simulink model "robot_stand"  (R2014b)
settings: Solver=ode45  StartTime=0.0  StopTime=10  FixedStep=1e-4  RelTol=1e-3
values from neighbouring files (symbols this model uses):
  robot_floor_friction_coeff = 0.6    [robot_init.m]
  robot_floor_position_gain = -1e5    (= -100000)    [robot_init.m]
  robot_floor_speed_gain = -1e3    (= -1000)    [robot_init.m]
  robot_gravity = [0 0 -9.80665]    [robot_init.m]
undefined symbols (not defined in the file or in its folder): CM730_acc_center, CM730_acc_gain, CM730_default, CM730_gyro_center, CM730_gyro_gain, CM730_sample_time, FSR_max, FSR_no_load, FSR_sample_time, FSR_scale, MX28_default, MX28_inertia, MX28_Te, X, Y, Z
libraries: sm_lib x158, fl_lib x128, nesl_utility x77
(part 1 of 6)
settings Model: BufferReuse=off  Creator=florent  LastModifiedBy=florent
settings DataIOCC: LimitDataPoints=off  SaveOutput=off  SignalLogging=off  DSMLogging=off  SaveTime=off
settings OptimizationCC: OptimizeBlockIOStorage=off  BufferReuse=off  GlobalBufferReuse=off  ExpressionFolding=off  LocalBlockOutputs=off
settings DebuggingCC: StateNameClashWarn=warning
settings DiagnosticsConfigSet: SimMechanicsConflictingReferenceFrames=none

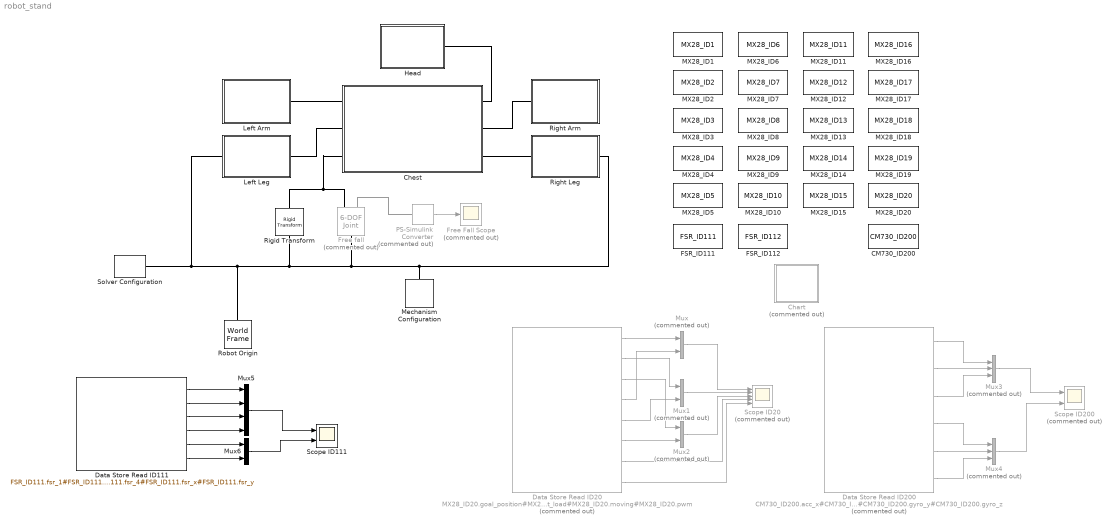
== system robot_stand ==
  CM730_ID200 : DataStoreMemory  DataStoreName=CM730_ID200  WriteAfterWriteMsg=error  InitialValue=CM730_default  VectorParams1D=off  OutDataTypeStr=Bus: CM730_bus
  Chart : Stateflow chart  Commented=on  TreatAsAtomicUnit=on
  Chest : Subsystem
      mask init:
      | [ModelDir,~,~] = fileparts(which(gcs));
      | 
      | Block = [gcb '/Solid'];
      | STLFileName = [ModelDir filesep 'STL' filesep 'Chest.STL'];
      | if ~strcmp(get_param(Block,'ExtGeomFileName'),STLFileName)
      |     set_param(Block,'ExtGeomFileName',STLFileName);
      | end
  Data Store Read ID111 : DataStoreRead  DataStoreName=FSR_ID111  SampleTime=MX28_Te  DataStoreElements=FSR_ID111.fsr_1#FSR_ID111.fsr_2#FSR_ID111.fsr_3#FSR_ID111.fsr_4#FSR_ID111.fsr_x#FSR_ID111.fsr_y
  Data Store Read ID20 : DataStoreRead  Commented=on  DataStoreName=MX28_ID20  SampleTime=MX28_Te  DataStoreElements=MX28_ID20.goal_position#MX28_ID20.moving_speed#MX28_ID20.torque_limit#MX28_ID20.present_position#MX28_ID20.present_speed#MX28_ID20.present_load#MX28_ID20.moving#MX28_ID20.pwm
  Data Store Read ID200 : DataStoreRead  Commented=on  DataStoreName=CM730_ID200  SampleTime=MX28_Te  DataStoreElements=CM730_ID200.acc_x#CM730_ID200.acc_y#CM730_ID200.acc_z#CM730_ID200.gyro_x#CM730_ID200.gyro_y#CM730_ID200.gyro_z
  FSR_ID111 : DataStoreMemory  DataStoreName=FSR_ID111  WriteAfterWriteMsg=error  InitialValue=FSR_default  VectorParams1D=off  OutDataTypeStr=Bus: FSR_bus
  FSR_ID112 : DataStoreMemory  DataStoreName=FSR_ID112  WriteAfterWriteMsg=error  InitialValue=FSR_default  VectorParams1D=off  OutDataTypeStr=Bus: FSR_bus
  Free Fall Scope : Scope  Commented=on
      settings: YMin=0.3418  YMax=0.34205  SaveName=ScopeData2
  Free fall : sm_lib/Joints/6-DOF Joint  Commented=on  SenseConstraintForce=off  SenseConstraintForceX=off  SenseConstraintForceY=off  SenseConstraintForceZ=off  SenseConstraintTorque=off  SenseConstraintTorqueX=off  SenseConstraintTorqueY=off  SenseConstraintTorqueZ=off  SenseTotalForce=off  SenseTotalForceX=off  SenseTotalForceY=off  SenseTotalForceZ=off  SenseTotalTorque=off  SenseTotalTorqueX=off  SenseTotalTorqueY=off  SenseTotalTorqueZ=off  CompositeWrenchDir=FollowerOnBase  CompositeWrenchFrame=BaseFrame  PxEquilibriumPosition=0  PxEquilibriumPositionUnits=m  PxSpringStiffness=0  PxSpringStiffnessUnits=N/m  PxDampingCoefficient=0  PxDampingCoefficientUnits=N/(m/s)  PxTorqueActuationMode=NoTorque  PxMotionActuationMode=ComputedMotion  PxSensePosition=off  PxSenseVelocity=off  PxSenseAcceleration=off  PxSenseTorqueForce=off  PxPositionTargetValue=0  PxPositionTargetValueUnits=m  PxPositionTargetSpecify=off  PxPositionTargetPriority=High  PxVelocityTargetValue=0  PxVelocityTargetValueUnits=m/s  PxVelocityTargetSpecify=off  PxVelocityTargetPriority=High  PyEquilibriumPosition=0  PyEquilibriumPositionUnits=m  PySpringStiffness=0  PySpringStiffnessUnits=N/m  PyDampingCoefficient=0  PyDampingCoefficientUnits=N/(m/s)  PyTorqueActuationMode=NoTorque  PyMotionActuationMode=ComputedMotion  PySensePosition=off  PySenseVelocity=off  PySenseAcceleration=off  PySenseTorqueForce=off  PyPositionTargetValue=0  PyPositionTargetValueUnits=m  PyPositionTargetSpecify=off  PyPositionTargetPriority=High  PyVelocityTargetValue=0  PyVelocityTargetValueUnits=m/s  PyVelocityTargetSpecify=off  PyVelocityTargetPriority=High  PzEquilibriumPosition=0  PzEquilibriumPositionUnits=m  PzSpringStiffness=0  PzSpringStiffnessUnits=N/m  PzDampingCoefficient=0  PzDampingCoefficientUnits=N/(m/s)  PzTorqueActuationMode=NoTorque  PzMotionActuationMode=ComputedMotion  PzSensePosition=on  PzSenseVelocity=off  PzSenseAcceleration=off  PzSenseTorqueForce=off  PzPositionTargetValue=342  PzPositionTargetValueUnits=mm  PzPositionTargetSpecify=on  PzPositionTargetPriority=High  PzVelocityTargetValue=0  PzVelocityTargetValueUnits=m/s  PzVelocityTargetSpecify=off  PzVelocityTargetPriority=High  SphDefPosRotationMethod=None  SphDefPosRotationAngleUnits=deg  SphDefPosRotationStandardAxis=+Z  SphDefPosRotationAngle=0.0  SphDefPosRotationArbitraryAxis=[0 0 1]  SphDefPosFollAlignAxisA=+X  SphDefPosBaseAlignAxisA=+Y  SphDefPosFollAlignAxisB=+Y  SphDefPosBaseAlignAxisB=+Z  SphDefPosRotationMatrix=[1 0 0; 0 1 0; 0 0 1]  SphEqPosRotationMethod=None  SphEqPosRotationAngleUnits=deg  SphEqPosRotationStandardAxis=+Z  SphEqPosRotationAngle=0.0  SphEqPosRotationArbitraryAxis=[0 0 1]  SphEqPosFollAlignAxisA=+X  SphEqPosBaseAlignAxisA=+Y  SphEqPosFollAlignAxisB=+Y  SphEqPosBaseAlignAxisB=+Z  SphEqPosRotationMatrix=[1 0 0; 0 1 0; 0 0 1]  SphSpringStiffness=0  SphSpringStiffnessUnits=N*m/deg  SphDampingCoefficient=0  SphDampingCoefficientUnits=N*m/(deg/s)  SphActuateTorqueX=off  SphActuateTorqueY=off  SphActuateTorqueZ=off  SphActuateTorque=off  SphTorqueActuationMode=NoTorque  SphMotionActuationMode=ComputedMotion  SphActuationFrame=BaseFrame  SphSensePosition=off  SphSenseVelocityX=off  SphSenseVelocityY=off  SphSenseVelocityZ=off  SphSenseVelocity=off  SphSenseAccelerationX=off  SphSenseAccelerationY=off  SphSenseAccelerationZ=off  SphSenseAcceleration=off  SphSenseTorqueX=off  SphSenseTorqueY=off  SphSenseTorqueZ=off  SphSenseTorqueForce=off  SphSensingFrame=BaseFrame  SphPositionTargetRotationMethod=None  SphPositionTargetRotationAngleUnits=deg  SphPositionTargetRotationStandardAxis=+Z  SphPositionTargetRotationAngle=0.0  SphPositionTargetRotationArbitraryAxis=[0 0 1]  SphPositionTargetFollAlignAxisA=+X  SphPositionTargetBaseAlignAxisA=+Y  SphPositionTargetFollAlignAxisB=+Y  SphPositionTargetBaseAlignAxisB=+Z  SphPositionTargetRotationMatrix=[1 0 0; 0 1 0; 0 0 1]  SphPositionTargetSpecify=off  SphPositionTargetPriority=High  SphVelocityTargetValue=[0 0 0]  SphVelocityTargetValueUnits=deg/s  SphVelocityTargetSpecify=off  SphVelocityTargetPriority=High  SphVelocityTargetInFollowerFrame=on  BlockFunction=simmechanics.library.joints.sixdof_joint
  Head : Subsystem
      mask init:
      | [ModelDir,~,~] = fileparts(which(gcs));
      | 
      | Block = [gcb '/Neck/Solid'];
      | STLFileName = [ModelDir filesep 'STL' filesep 'Neck.STL'];
      | if ~strcmp(get_param(Block,'ExtGeomFileName'),STLFileName)
      |     set_param(Block,'ExtGeomFileName',STLFileName);
      | end
      | 
      | Block = [gcb '/Head/Solid'];
      | STLFileName = [ModelDir filesep 'STL' filesep 'Head.STL'];
      | if ~strcmp(get_param(Block,'ExtGeomFileName'),STLFileName)
      |     set_param(Block,'ExtGeomFileName',STLFileName);
      | end
  Left Arm : Subsystem
      mask init:
      | [ModelDir,~,~] = fileparts(which(gcs));
      | 
      | Block = [gcb '/Left Shoulder/Solid'];
      | STLFileName = [ModelDir filesep 'STL' filesep 'Left_shoulder.STL'];
      | if ~strcmp(get_param(Block,'ExtGeomFileName'),STLFileName)
      |     set_param(Block,'ExtGeomFileName',STLFileName);
      | end
      | 
      | Block = [gcb '/Left Upper Arm/Solid'];
      | STLFileName = [ModelDir filesep 'STL' filesep 'Left_Arm.STL'];
      | if ~strcmp(get_param(Block,'ExtGeomFileName'),STLFileName)
      |     set_param(Block,'ExtGeomFileName',STLFileName);
      | end
      | 
      | Block = [gcb '/Left Forearm/Solid'];
      | STLFileName = [ModelDir filesep 'STL' filesep 'Left_Forearm.STL'];
      | if ~strcmp(get_param(Block,'ExtGeomFileName'),STLFileName)
      |     set_param(Block,'ExtGeomFileName',STLFileName);
      | end
  Left Leg : Subsystem
      mask init:
      | [ModelDir,~,~] = fileparts(which(gcs));
      | 
      | Block = [gcb '/Left Hip Yaw/Solid'];
      | STLFileName = [ModelDir filesep 'STL' filesep 'Hip1.STL'];
      | if ~strcmp(get_param(Block,'ExtGeomFileName'),STLFileName)
      |     set_param(Block,'ExtGeomFileName',STLFileName);
      | end
      | 
      | Block = [gcb '/Left Hip Roll/Solid'];
      | STLFileName = [ModelDir filesep 'STL' filesep 'Left_Hip2.STL'];
      | if ~strcmp(get_param(Block,'ExtGeomFileName'),STLFileName)
      |     set_param(Block,'ExtGeomFileName',STLFileName);
      | end
      | 
      | Block = [gcb '/Left Thigh/Solid'];
      | STLFileName = [ModelDir filesep 'STL' filesep 'Left_Thigh.STL'];
      | if ~strcmp(get_param(Block,'ExtGeomFileName'),STLFileName)
      |     set_param(Block,'ExtGeomFileName',STLFileName);
      | end
      | 
      | Block = [gcb '/Left Lower Leg/Solid'];
      | STLFileName = [ModelDir filesep 'STL' filesep 'Left_Lower_Leg.STL'];
      | if ~strcmp(get_param(Block,'ExtGeomFileName'),STLFileName)
      |     set_param(Block,'ExtGeomFileName',STLFileName);
      | end
      | 
      | Block = [gcb '/Left Ankle/Solid'];
      | STLFileName = [ModelDir filesep 'STL' filesep 'Left_Ankle.STL'];
      | if ~strcmp(get_param(Block,'ExtGeomFileName'),STLFileName)
      |     set_param(Block,'ExtGeomFileName',STLFileName);
      | end
      | 
      | Block = [gcb '/Left Foot/Solid'];
      | STLFileName = [ModelDir filesep 'STL' filesep 'Left_Foot.STL'];
      | if ~strcmp(get_param(Block,'ExtGeomFileName'),STLFileName)
      |     set_param(Block,'ExtGeomFileName',STLFileName);
      | end
  MX28_ID1 : DataStoreMemory  DataStoreName=MX28_ID1  WriteAfterWriteMsg=error  InitialValue=MX28_default  VectorParams1D=off  OutDataTypeStr=Bus: MX28_bus
  MX28_ID10 : DataStoreMemory  DataStoreName=MX28_ID10  WriteAfterWriteMsg=error  InitialValue=MX28_default  VectorParams1D=off  OutDataTypeStr=Bus: MX28_bus
  MX28_ID11 : DataStoreMemory  DataStoreName=MX28_ID11  WriteAfterWriteMsg=error  InitialValue=MX28_default  VectorParams1D=off  OutDataTypeStr=Bus: MX28_bus
  MX28_ID12 : DataStoreMemory  DataStoreName=MX28_ID12  WriteAfterWriteMsg=error  InitialValue=MX28_default  VectorParams1D=off  OutDataTypeStr=Bus: MX28_bus
  MX28_ID13 : DataStoreMemory  DataStoreName=MX28_ID13  WriteAfterWriteMsg=error  InitialValue=MX28_default  VectorParams1D=off  OutDataTypeStr=Bus: MX28_bus
  MX28_ID14 : DataStoreMemory  DataStoreName=MX28_ID14  WriteAfterWriteMsg=error  InitialValue=MX28_default  VectorParams1D=off  OutDataTypeStr=Bus: MX28_bus
  MX28_ID15 : DataStoreMemory  DataStoreName=MX28_ID15  WriteAfterWriteMsg=error  InitialValue=MX28_default  VectorParams1D=off  OutDataTypeStr=Bus: MX28_bus
  MX28_ID16 : DataStoreMemory  DataStoreName=MX28_ID16  WriteAfterWriteMsg=error  InitialValue=MX28_default  VectorParams1D=off  OutDataTypeStr=Bus: MX28_bus
  MX28_ID17 : DataStoreMemory  DataStoreName=MX28_ID17  WriteAfterWriteMsg=error  InitialValue=MX28_default  VectorParams1D=off  OutDataTypeStr=Bus: MX28_bus
  MX28_ID18 : DataStoreMemory  DataStoreName=MX28_ID18  WriteAfterWriteMsg=error  InitialValue=MX28_default  VectorParams1D=off  OutDataTypeStr=Bus: MX28_bus
  MX28_ID19 : DataStoreMemory  DataStoreName=MX28_ID19  WriteAfterWriteMsg=error  InitialValue=MX28_default  VectorParams1D=off  OutDataTypeStr=Bus: MX28_bus
  MX28_ID2 : DataStoreMemory  DataStoreName=MX28_ID2  WriteAfterWriteMsg=error  InitialValue=MX28_default  VectorParams1D=off  OutDataTypeStr=Bus: MX28_bus
  MX28_ID20 : DataStoreMemory  DataStoreName=MX28_ID20  WriteAfterWriteMsg=error  InitialValue=MX28_default  VectorParams1D=off  OutDataTypeStr=Bus: MX28_bus
  MX28_ID3 : DataStoreMemory  DataStoreName=MX28_ID3  WriteAfterWriteMsg=error  InitialValue=MX28_default  VectorParams1D=off  OutDataTypeStr=Bus: MX28_bus
  MX28_ID4 : DataStoreMemory  DataStoreName=MX28_ID4  WriteAfterWriteMsg=error  InitialValue=MX28_default  VectorParams1D=off  OutDataTypeStr=Bus: MX28_bus
  MX28_ID5 : DataStoreMemory  DataStoreName=MX28_ID5  WriteAfterWriteMsg=error  InitialValue=MX28_default  VectorParams1D=off  OutDataTypeStr=Bus: MX28_bus
  MX28_ID6 : DataStoreMemory  DataStoreName=MX28_ID6  WriteAfterWriteMsg=error  InitialValue=MX28_default  VectorParams1D=off  OutDataTypeStr=Bus: MX28_bus
  MX28_ID7 : DataStoreMemory  DataStoreName=MX28_ID7  WriteAfterWriteMsg=error  InitialValue=MX28_default  VectorParams1D=off  OutDataTypeStr=Bus: MX28_bus
  MX28_ID8 : DataStoreMemory  DataStoreName=MX28_ID8  WriteAfterWriteMsg=error  InitialValue=MX28_default  VectorParams1D=off  OutDataTypeStr=Bus: MX28_bus
  MX28_ID9 : DataStoreMemory  DataStoreName=MX28_ID9  WriteAfterWriteMsg=error  InitialValue=MX28_default  VectorParams1D=off  OutDataTypeStr=Bus: MX28_bus
  Mechanism Configuration : sm_lib/Utilities/Mechanism Configuration  UniformGravity=Constant  GravityVector=robot_gravity  GravityUnits=m/s^2  LinearizationDelta=0.001  BlockFunction=simmechanics.library.utilities.mechanism_configuration
  Mux : Mux  Commented=on  Inputs=2
  Mux1 : Mux  Commented=on  Inputs=2
  Mux2 : Mux  Commented=on  Inputs=2
  Mux3 : Mux  Commented=on  Inputs=3
  Mux4 : Mux  Commented=on  Inputs=3
  Mux5 : Mux
  Mux6 : Mux  Inputs=2
  PS-Simulink Converter : nesl_utility/PS-Simulink Converter  Commented=on  PhysicalDomain=network_engine_domain  SubClassName=ps_output  LeftPortType=input  RightPortType=output  PseudoPeriodic=off  Frequencies=[]  Unit=m  AffineConversion=off
  Right Arm : Subsystem
      mask init:
      | [ModelDir,~,~] = fileparts(which(gcs));
      | 
      | Block = [gcb '/Right Shoulder/Solid'];
      | STLFileName = [ModelDir filesep 'STL' filesep 'Right_shoulder.STL'];
      | if ~strcmp(get_param(Block,'ExtGeomFileName'),STLFileName)
      |     set_param(Block,'ExtGeomFileName',STLFileName);
      | end
      | 
      | Block = [gcb '/Right Upper Arm/Solid'];
      | STLFileName = [ModelDir filesep 'STL' filesep 'Right_Arm.STL'];
      | if ~strcmp(get_param(Block,'ExtGeomFileName'),STLFileName)
      |     set_param(Block,'ExtGeomFileName',STLFileName);
      | end
      | 
      | Block = [gcb '/Right Forearm/Solid'];
      | STLFileName = [ModelDir filesep 'STL' filesep 'Right_Forearm.STL'];
      | if ~strcmp(get_param(Block,'ExtGeomFileName'),STLFileName)
      |     set_param(Block,'ExtGeomFileName',STLFileName);
      | end
  Right Leg : Subsystem
      mask init:
      | [ModelDir,~,~] = fileparts(which(gcs));
      | 
      | Block = [gcb '/Right Hip Yaw/Solid'];
      | STLFileName = [ModelDir filesep 'STL' filesep 'Hip1.STL'];
      | if ~strcmp(get_param(Block,'ExtGeomFileName'),STLFileName)
      |     set_param(Block,'ExtGeomFileName',STLFileName);
      | end
      | 
      | Block = [gcb '/Right Hip Roll/Solid'];
      | STLFileName = [ModelDir filesep 'STL' filesep 'Right_Hip2.STL'];
      | if ~strcmp(get_param(Block,'ExtGeomFileName'),STLFileName)
      |     set_param(Block,'ExtGeomFileName',STLFileName);
      | end
      | 
      | Block = [gcb '/Right Thigh/Solid'];
      | STLFileName = [ModelDir filesep 'STL' filesep 'Right_Thigh.STL'];
      | if ~strcmp(get_param(Block,'ExtGeomFileName'),STLFileName)
      |     set_param(Block,'ExtGeomFileName',STLFileName);
      | end
      | 
      | Block = [gcb '/Right Lower Leg/Solid'];
      | STLFileName = [ModelDir filesep 'STL' filesep 'Right_Lower_Leg.STL'];
      | if ~strcmp(get_param(Block,'ExtGeomFileName'),STLFileName)
      |     set_param(Block,'ExtGeomFileName',STLFileName);
      | end
      | 
      | Block = [gcb '/Right Ankle/Solid'];
      | STLFileName = [ModelDir filesep 'STL' filesep 'Right_Ankle.STL'];
      | if ~strcmp(get_param(Block,'ExtGeomFileName'),STLFileName)
      |     set_param(Block,'ExtGeomFileName',STLFileName);
      | end
      | 
      | Block = [gcb '/Right Foot/Solid'];
      | STLFileName = [ModelDir filesep 'STL' filesep 'Right_Foot.STL'];
      | if ~strcmp(get_param(Block,'ExtGeomFileName'),STLFileName)
      |     set_param(Block,'ExtGeomFileName',STLFileName);
      | end
  Rigid Transform : sm_lib/Frames and Transforms/Rigid Transform  TranslationMethod=Cartesian  TranslationLengthUnit=mm  TranslationStandardAxis=+Z  TranslationStandardOffset=0  TranslationCartesianOffset=[0 0 500]  TranslationROffset=0  TranslationROffsetUnits=m  TranslationZOffset=0  TranslationZOffsetUnits=m  TranslationThetaOffset=0  TranslationThetaOffsetUnits=deg  RotationMethod=None  RotationAngleUnits=deg  RotationStandardAxis=+Z  RotationAngle=0.0  RotationArbitraryAxis=[0 0 1]  FollAlignAxisA=+X  BaseAlignAxisA=+Y  FollAlignAxisB=+Y  BaseAlignAxisB=+Z  RotationMatrix=[1 0 0; 0 1 0; 0 0 1]  BlockFunction=simmechanics.library.frames_transforms.rigid_transform
  Robot Origin : sm_lib/Frames and Transforms/World Frame  BlockFunction=simmechanics.library.frames_transforms.world_frame
  Scope ID111 : Scope  NumInputPorts=2
      settings: YMin=-1~254  YMax=1~256  SaveName=ScopeData3
  Scope ID20 : Scope  Commented=on  NumInputPorts=5
      settings: YMin=1825~-250~-1250~-5~-5  YMax=2250~350~1250~5~5
  Scope ID200 : Scope  Commented=on  NumInputPorts=2
      settings: YMin=0~510  YMax=1200~512
  Solver Configuration : nesl_utility/Solver Configuration  PhysicalDomain=network_engine_domain  SubClassName=solver  LeftPortType=input  RightPortType=generic  Accelerate=off  Tones=[]  Harmonics=[]  SimulateNoise=off  Profile=off  UseLocalSampling=off  EnableSwitchedLinearOptims=on  FrequencyDomain=off  UseCCode=off  RelTol=0.001  AbsTol=1e-06  MinStep=1e-09  ToWorkspace=off  DoDC=off  ResidualTolerance=1e-05  UseLocalSolver=off  LocalSolverChoice=NE_BACKWARD_EULER_ADVANCER  LocalSolverSampleTime=0.0001  DoFixedCost=off  MaxNonlinIter=3  MaxModeIter=2  LinearAlgebra=Sparse  DelaysMemoryBudget=1024  AutomaticFiltering=on  FilteringTimeConstant=0.001
  wires:
  Mux/1 -> Scope ID20/1
  Mux1/1 -> Scope ID20/2
  Mux2/1 -> Scope ID20/3
  Data Store Read ID20/6 -> Mux2/2
  Data Store Read ID20/5 -> Mux1/2
  Data Store Read ID20/4 -> Mux/2
  Data Store Read ID20/3 -> Mux2/1
  Data Store Read ID20/2 -> Mux1/1
  Data Store Read ID20/1 -> Mux/1
  Data Store Read ID20/8 -> Scope ID20/5
  Data Store Read ID20/7 -> Scope ID20/4
  Mux3/1 -> Scope ID200/1
  Mux4/1 -> Scope ID200/2
  Data Store Read ID200/2 -> Mux3/2
  Data Store Read ID200/1 -> Mux3/1
  Data Store Read ID200/3 -> Mux3/3
  Data Store Read ID200/4 -> Mux4/1
  Data Store Read ID200/5 -> Mux4/2
  Data Store Read ID200/6 -> Mux4/3
  PS-Simulink Converter/1 -> Free Fall Scope/1
  Mux6/1 -> Scope ID111/2
  Data Store Read ID111/5 -> Mux6/1
  Data Store Read ID111/6 -> Mux6/2
  Data Store Read ID111/1 -> Mux5/1
  Data Store Read ID111/2 -> Mux5/2
  Data Store Read ID111/4 -> Mux5/4
  Data Store Read ID111/3 -> Mux5/3
  Mux5/1 -> Scope ID111/1
  connections:
  Head/LConn1 -- Chest/RConn1
  Chest/RConn2 -- Right Arm/LConn1
  Left Arm/RConn1 -- Chest/LConn1
  Right Leg/LConn1 -- Chest/RConn3
  Left Leg/RConn1 -- Chest/LConn2
  Solver Configuration/RConn1 -- Left Leg/LConn1 -- Right Leg/RConn1 -- Mechanism Configuration/RConn1 -- Free fall/LConn1 -- Rigid Transform/LConn1 -- Robot Origin/RConn1
  Rigid Transform/RConn1 -- Free fall/RConn1 -- Chest/LConn3
  PS-Simulink Converter/LConn1 -- Free fall/RConn2

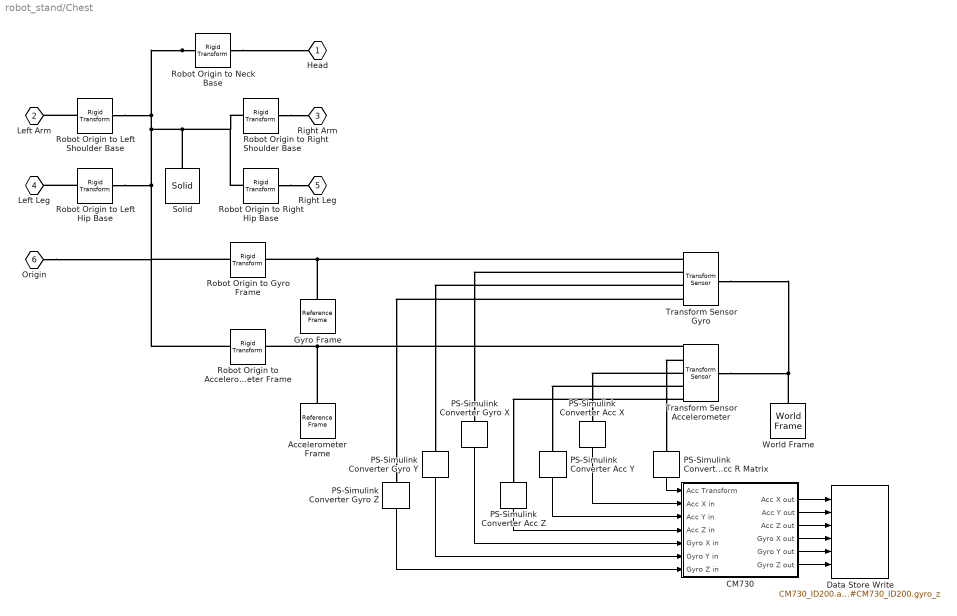
== system robot_stand/Chest ==
  Accelerometer Frame : sm_lib/Frames and Transforms/Reference Frame  BlockFunction=simmechanics.library.frames_transforms.reference_frame
  CM730 : Subsystem  TreatAsAtomicUnit=on  SystemSampleTime=CM730_sample_time
  Data Store Write : DataStoreWrite  DataStoreName=CM730_ID200  DataStoreElements=CM730_ID200.acc_x#CM730_ID200.acc_y#CM730_ID200.acc_z#CM730_ID200.gyro_x#CM730_ID200.gyro_y#CM730_ID200.gyro_z
  Gyro Frame : sm_lib/Frames and Transforms/Reference Frame  BlockFunction=simmechanics.library.frames_transforms.reference_frame
  PS-Simulink Converter Acc R Matrix : nesl_utility/PS-Simulink Converter  PhysicalDomain=network_engine_domain  SubClassName=ps_output  LeftPortType=input  RightPortType=output  PseudoPeriodic=off  Frequencies=[]  Unit=1  AffineConversion=off
  PS-Simulink Converter Acc X : nesl_utility/PS-Simulink Converter  PhysicalDomain=network_engine_domain  SubClassName=ps_output  LeftPortType=input  RightPortType=output  PseudoPeriodic=off  Frequencies=[]  Unit=m/s^2  AffineConversion=off
  PS-Simulink Converter Acc Y : nesl_utility/PS-Simulink Converter  PhysicalDomain=network_engine_domain  SubClassName=ps_output  LeftPortType=input  RightPortType=output  PseudoPeriodic=off  Frequencies=[]  Unit=m/s^2  AffineConversion=off
  PS-Simulink Converter Acc Z : nesl_utility/PS-Simulink Converter  PhysicalDomain=network_engine_domain  SubClassName=ps_output  LeftPortType=input  RightPortType=output  PseudoPeriodic=off  Frequencies=[]  Unit=m/s^2  AffineConversion=off
  PS-Simulink Converter Gyro X : nesl_utility/PS-Simulink Converter  PhysicalDomain=network_engine_domain  SubClassName=ps_output  LeftPortType=input  RightPortType=output  PseudoPeriodic=off  Frequencies=[]  Unit=rad/s  AffineConversion=off
  PS-Simulink Converter Gyro Y : nesl_utility/PS-Simulink Converter  PhysicalDomain=network_engine_domain  SubClassName=ps_output  LeftPortType=input  RightPortType=output  PseudoPeriodic=off  Frequencies=[]  Unit=rad/s  AffineConversion=off
  PS-Simulink Converter Gyro Z : nesl_utility/PS-Simulink Converter  PhysicalDomain=network_engine_domain  SubClassName=ps_output  LeftPortType=input  RightPortType=output  PseudoPeriodic=off  Frequencies=[]  Unit=rad/s  AffineConversion=off
  Robot Origin to Accelerometer Frame : sm_lib/Frames and Transforms/Rigid Transform  TranslationMethod=Cartesian  TranslationLengthUnit=mm  TranslationStandardAxis=+Z  TranslationStandardOffset=0  TranslationCartesianOffset=[0 -10 -31.6]  TranslationROffset=0  TranslationROffsetUnits=m  TranslationZOffset=0  TranslationZOffsetUnits=m  TranslationThetaOffset=0  TranslationThetaOffsetUnits=deg  RotationMethod=None  RotationAngleUnits=deg  RotationStandardAxis=+Z  RotationAngle=0  RotationArbitraryAxis=[0 0 1]  FollAlignAxisA=+X  BaseAlignAxisA=-Y  FollAlignAxisB=+Z  BaseAlignAxisB=+Z  RotationMatrix=[1 0 0; 0 1 0; 0 0 1]  BlockFunction=simmechanics.library.frames_transforms.rigid_transform
  Robot Origin to Gyro Frame : sm_lib/Frames and Transforms/Rigid Transform  TranslationMethod=Cartesian  TranslationLengthUnit=mm  TranslationStandardAxis=+Z  TranslationStandardOffset=0  TranslationCartesianOffset=[0 10 -31.6]  TranslationROffset=0  TranslationROffsetUnits=m  TranslationZOffset=0  TranslationZOffsetUnits=m  TranslationThetaOffset=0  TranslationThetaOffsetUnits=deg  RotationMethod=AlignedAxes  RotationAngleUnits=deg  RotationStandardAxis=+Z  RotationAngle=0  RotationArbitraryAxis=[0 0 1]  FollAlignAxisA=+X  BaseAlignAxisA=-Y  FollAlignAxisB=+Z  BaseAlignAxisB=-Z  RotationMatrix=[1 0 0; 0 1 0; 0 0 1]  BlockFunction=simmechanics.library.frames_transforms.rigid_transform
  Robot Origin to Left Hip Base : sm_lib/Frames and Transforms/Rigid Transform  TranslationMethod=Cartesian  TranslationLengthUnit=mm  TranslationStandardAxis=+Z  TranslationStandardOffset=0  TranslationCartesianOffset=[37 5 -94.2]  TranslationROffset=0  TranslationROffsetUnits=m  TranslationZOffset=0  TranslationZOffsetUnits=m  TranslationThetaOffset=0  TranslationThetaOffsetUnits=deg  RotationMethod=AlignedAxes  RotationAngleUnits=deg  RotationStandardAxis=+Z  RotationAngle=0  RotationArbitraryAxis=[0 0 1]  FollAlignAxisA=+X  BaseAlignAxisA=-Y  FollAlignAxisB=+Y  BaseAlignAxisB=-X  RotationMatrix=[1 0 0; 0 1 0; 0 0 1]  BlockFunction=simmechanics.library.frames_transforms.rigid_transform
  Robot Origin to Left Shoulder Base : sm_lib/Frames and Transforms/Rigid Transform  TranslationMethod=Cartesian  TranslationLengthUnit=mm  TranslationStandardAxis=+Z  TranslationStandardOffset=0  TranslationCartesianOffset=[60.9 0 0.1]  TranslationROffset=0  TranslationROffsetUnits=m  TranslationZOffset=0  TranslationZOffsetUnits=m  TranslationThetaOffset=0  TranslationThetaOffsetUnits=deg  RotationMethod=AlignedAxes  RotationAngleUnits=deg  RotationStandardAxis=+Z  RotationAngle=0  RotationArbitraryAxis=[0 0 1]  FollAlignAxisA=+X  BaseAlignAxisA=+Y  FollAlignAxisB=+Y  BaseAlignAxisB=+Z  RotationMatrix=[1 0 0; 0 1 0; 0 0 1]  BlockFunction=simmechanics.library.frames_transforms.rigid_transform
  Robot Origin to Neck Base : sm_lib/Frames and Transforms/Rigid Transform  TranslationMethod=Cartesian  TranslationLengthUnit=mm  TranslationStandardAxis=+Z  TranslationStandardOffset=0  TranslationCartesianOffset=[0 0 23.9]  TranslationROffset=0  TranslationROffsetUnits=m  TranslationZOffset=0  TranslationZOffsetUnits=m  TranslationThetaOffset=0  TranslationThetaOffsetUnits=deg  RotationMethod=None  RotationAngleUnits=deg  RotationStandardAxis=+Z  RotationAngle=0  RotationArbitraryAxis=[0 0 1]  FollAlignAxisA=+X  BaseAlignAxisA=+Y  FollAlignAxisB=+Y  BaseAlignAxisB=+Z  RotationMatrix=[1 0 0; 0 1 0; 0 0 1]  BlockFunction=simmechanics.library.frames_transforms.rigid_transform
  Robot Origin to Right Hip Base : sm_lib/Frames and Transforms/Rigid Transform  TranslationMethod=Cartesian  TranslationLengthUnit=mm  TranslationStandardAxis=+Z  TranslationStandardOffset=0  TranslationCartesianOffset=[-37 5 -94.2]  TranslationROffset=0  TranslationROffsetUnits=m  TranslationZOffset=0  TranslationZOffsetUnits=m  TranslationThetaOffset=0  TranslationThetaOffsetUnits=deg  RotationMethod=AlignedAxes  RotationAngleUnits=deg  RotationStandardAxis=+Z  RotationAngle=0  RotationArbitraryAxis=[0 0 1]  FollAlignAxisA=+X  BaseAlignAxisA=-Y  FollAlignAxisB=+Y  BaseAlignAxisB=-X  RotationMatrix=[1 0 0; 0 1 0; 0 0 1]  BlockFunction=simmechanics.library.frames_transforms.rigid_transform
  Robot Origin to Right Shoulder Base : sm_lib/Frames and Transforms/Rigid Transform  TranslationMethod=Cartesian  TranslationLengthUnit=mm  TranslationStandardAxis=+Z  TranslationStandardOffset=0  TranslationCartesianOffset=[-60.90 0 0.1]  TranslationROffset=0  TranslationROffsetUnits=m  TranslationZOffset=0  TranslationZOffsetUnits=m  TranslationThetaOffset=0  TranslationThetaOffsetUnits=deg  RotationMethod=AlignedAxes  RotationAngleUnits=deg  RotationStandardAxis=+Z  RotationAngle=0  RotationArbitraryAxis=[0 0 1]  FollAlignAxisA=-Z  BaseAlignAxisA=+X  FollAlignAxisB=-X  BaseAlignAxisB=+Y  RotationMatrix=[1 0 0; 0 1 0; 0 0 1]  BlockFunction=simmechanics.library.frames_transforms.rigid_transform
  Solid : sm_lib/Body Elements/Solid  InertiaType=Custom  Mass=591.6  MassUnits=g  CenterOfMass=[0.06 16.94 -31.61]  CenterOfMassUnits=mm  MomentsOfInertia=[487010 528783 581903]  MomentsOfInertiaUnits=g*mm^2  ProductsOfInertia=[17259 -433 351]  ProductsOfInertiaUnits=g*mm^2  DensityBased=on  Density=1000  DensityUnits=kg/(m^3)  GraphicType=FromGeometry  MarkerShape=Sphere  MarkerSize=10  MarkerSizeUnits=m  GraphicVisPropType=SimpleVisualProperties  GraphicDiffuseColor=[0.5 0.5 0.5]  GraphicSpecularColor=[0.5 0.5 0.5 1.0]  GraphicAmbientColor=[0.15 0.15 0.15 1.0]  GraphicEmissiveColor=[0.0 0.0 0.0 1.0]  GraphicShininess=75  GraphicOpacity=1.0  GeometryShape=FromFile  RectangleSize=[1 1]  RectangleSizeUnits=m  BrickDimensions=[115.5 112.1 47.8]  BrickDimensionUnits=mm  CylinderRadius=1  CylinderRadiusUnits=m  CylinderLength=1  CylinderLengthUnits=m  SphereRadius=1  SphereRadiusUnits=m  EllipsoidRadii=[1 1 1]  EllipsoidRadiiUnits=m  ExtrusionCrossSection=[1 1; -1 1; -1 -1; 1 -1]  ExtrusionCrossSectionUnits=m  ExtrusionLength=1  ExtrusionLengthUnits=m  PolygonNumSides=3  PolygonOuterRadius=1  PolygonOuterRadiusUnits=m  ExtGeomFileType=STL  ExtGeomFileName=D:\Ker Lann\systemes\darwin\kinematics\STL\Chest.STL  ExtGeomFileUnits=mm  RevolutionCrossSection=[1 1; 1 -1; 2 -1; 2 1]  RevolutionCrossSectionUnits=m  RevolutionExtent=Full  RevolutionAngle=180  RevolutionAngleUnits=deg  BlockFunction=simmechanics.library.body_elements.solid
  Transform Sensor Accelerometer : sm_lib/Frames and Transforms/Transform Sensor  MeasurementFrame=Follower  SenseAngle=off  SenseAxis=off  SenseAngle1=off  SenseAngle2=off  SenseAngle3=off  SenseQ=off  SenseR=on  SenseOmegaX=off  SenseOmegaY=off  SenseOmegaZ=off  SenseOmega1=off  SenseOmega2=off  SenseOmega3=off  SenseQDot=off  SenseRDot=off  SenseAlphaX=off  SenseAlphaY=off  SenseAlphaZ=off  SenseAlpha1=off  SenseAlpha2=off  SenseAlpha3=off  SenseQDDot=off  SenseRDDot=off  SenseX=off  SenseY=off  SenseZ=off  SenseRad=off  SenseAzim=off  SenseDist=off  SenseInc=off  SenseXDot=off  SenseYDot=off  SenseZDot=off  SenseRadDot=off  SenseAzimDot=off  SenseDistDot=off  SenseIncDot=off  SenseXDDot=on  SenseYDDot=on  SenseZDDot=on  SenseRadDDot=off  SenseAzimDDot=off  SenseDistDDot=off  SenseIncDDot=off  BlockFunction=simmechanics.library.frames_transforms.transform_sensor
  Transform Sensor Gyro : sm_lib/Frames and Transforms/Transform Sensor  MeasurementFrame=Follower  SenseAngle=off  SenseAxis=off  SenseAngle1=off  SenseAngle2=off  SenseAngle3=off  SenseQ=off  SenseR=off  SenseOmegaX=on  SenseOmegaY=on  SenseOmegaZ=on  SenseOmega1=off  SenseOmega2=off  SenseOmega3=off  SenseQDot=off  SenseRDot=off  SenseAlphaX=off  SenseAlphaY=off  SenseAlphaZ=off  SenseAlpha1=off  SenseAlpha2=off  SenseAlpha3=off  SenseQDDot=off  SenseRDDot=off  SenseX=off  SenseY=off  SenseZ=off  SenseRad=off  SenseAzim=off  SenseDist=off  SenseInc=off  SenseXDot=off  SenseYDot=off  SenseZDot=off  SenseRadDot=off  SenseAzimDot=off  SenseDistDot=off  SenseIncDot=off  SenseXDDot=off  SenseYDDot=off  SenseZDDot=off  SenseRadDDot=off  SenseAzimDDot=off  SenseDistDDot=off  SenseIncDDot=off  BlockFunction=simmechanics.library.frames_transforms.transform_sensor
  World Frame : sm_lib/Frames and Transforms/World Frame  BlockFunction=simmechanics.library.frames_transforms.world_frame
  Head : PMIOPort  Port=1  Side=Right
  Left Arm : PMIOPort  Port=2  Side=Left
  Right Arm : PMIOPort  Port=3  Side=Right
  Left Leg : PMIOPort  Port=4  Side=Left
  Right Leg : PMIOPort  Port=5  Side=Right
  Origin : PMIOPort  Port=6  Side=Left
  wires:
  CM730/1(Acc X out) -> Data Store Write/1
  CM730/2(Acc Y out) -> Data Store Write/2
  CM730/3(Acc Z out) -> Data Store Write/3
  CM730/4(Gyro X out) -> Data Store Write/4
  CM730/5(Gyro Y out) -> Data Store Write/5
  CM730/6(Gyro Z out) -> Data Store Write/6
  PS-Simulink Converter Acc X/1 -> CM730/2(Acc X in)
  PS-Simulink Converter Acc Y/1 -> CM730/3(Acc Y in)
  PS-Simulink Converter Acc Z/1 -> CM730/4(Acc Z in)
  PS-Simulink Converter Gyro X/1 -> CM730/5(Gyro X in)
  PS-Simulink Converter Gyro Z/1 -> CM730/7(Gyro Z in)
  PS-Simulink Converter Gyro Y/1 -> CM730/6(Gyro Y in)
  PS-Simulink Converter Acc R Matrix/1 -> CM730/1(Acc Transform)
  connections:
  Robot Origin to Neck Base/RConn1 -- Head/RConn1
  Robot Origin to Right Shoulder Base/RConn1 -- Right Arm/RConn1
  Robot Origin to Right Hip Base/RConn1 -- Right Leg/RConn1
  Robot Origin to Neck Base/LConn1 -- Robot Origin to Left Shoulder Base/LConn1 -- Robot Origin to Accelerometer Frame/LConn1 -- Origin/RConn1 -- Robot Origin to Gyro Frame/LConn1 -- Robot Origin to Left Hip Base/LConn1 -- Robot Origin to Right Hip Base/LConn1 -- Robot Origin to Right Shoulder Base/LConn1 -- Solid/RConn1
  Robot Origin to Left Shoulder Base/RConn1 -- Left Arm/RConn1
  Robot Origin to Left Hip Base/RConn1 -- Left Leg/RConn1
  Gyro Frame/RConn1 -- Transform Sensor Gyro/RConn1 -- Robot Origin to Gyro Frame/RConn1
  Accelerometer Frame/RConn1 -- Transform Sensor Accelerometer/RConn1 -- Robot Origin to Accelerometer Frame/RConn1
  World Frame/RConn1 -- Transform Sensor Gyro/LConn1 -- Transform Sensor Accelerometer/LConn1
  Transform Sensor Gyro/RConn2 -- PS-Simulink Converter Gyro X/LConn1
  Transform Sensor Gyro/RConn3 -- PS-Simulink Converter Gyro Y/LConn1
  Transform Sensor Gyro/RConn4 -- PS-Simulink Converter Gyro Z/LConn1
  Transform Sensor Accelerometer/RConn2 -- PS-Simulink Converter Acc R Matrix/LConn1
  Transform Sensor Accelerometer/RConn5 -- PS-Simulink Converter Acc Z/LConn1
  Transform Sensor Accelerometer/RConn4 -- PS-Simulink Converter Acc Y/LConn1
  Transform Sensor Accelerometer/RConn3 -- PS-Simulink Converter Acc X/LConn1

== system robot_stand/Head ==
  Head : Subsystem
  Head Axis : sm_lib/Frames and Transforms/Reference Frame  BlockFunction=simmechanics.library.frames_transforms.reference_frame
  Head Origin : sm_lib/Frames and Transforms/Reference Frame  BlockFunction=simmechanics.library.frames_transforms.reference_frame
  Head Pan (19) : Subsystem
  Head Tilt (20) : Subsystem
  Neck : Subsystem
  Neck Axis : sm_lib/Frames and Transforms/Reference Frame  BlockFunction=simmechanics.library.frames_transforms.reference_frame
  Neck Base : sm_lib/Frames and Transforms/Reference Frame  BlockFunction=simmechanics.library.frames_transforms.reference_frame
  Chest : PMIOPort  Port=1  Side=Left
  connections:
  Neck Axis/RConn1 -- Head Pan (19)/RConn1 -- Neck/LConn1
  Neck Base/RConn1 -- Head Pan (19)/LConn1 -- Chest/RConn1
  Neck/RConn1 -- Head Tilt (20)/LConn1 -- Head Origin/RConn1
  Head/LConn1 -- Head Tilt (20)/RConn1 -- Head Axis/RConn1

== system robot_stand/Left Arm ==
  Left Arm Axis : sm_lib/Frames and Transforms/Reference Frame  BlockFunction=simmechanics.library.frames_transforms.reference_frame
  Left Arm Base : sm_lib/Frames and Transforms/Reference Frame  BlockFunction=simmechanics.library.frames_transforms.reference_frame
  Left Elbow (6) : Subsystem
  Left Forearm : Subsystem
  Left Forearm Axis : sm_lib/Frames and Transforms/Reference Frame  BlockFunction=simmechanics.library.frames_transforms.reference_frame
  Left Forearm Base : sm_lib/Frames and Transforms/Reference Frame  BlockFunction=simmechanics.library.frames_transforms.reference_frame
  Left Shoulder : Subsystem
  Left Shoulder Axis : sm_lib/Frames and Transforms/Reference Frame  BlockFunction=simmechanics.library.frames_transforms.reference_frame
  Left Shoulder Base : sm_lib/Frames and Transforms/Reference Frame  BlockFunction=simmechanics.library.frames_transforms.reference_frame
  Left Shoulder Pitch (2) : Subsystem
  Left Shoulder Roll (4) : Subsystem
  Left Upper Arm : Subsystem
  Chest : PMIOPort  Port=1  Side=Right
  connections:
  Chest/RConn1 -- Left Shoulder Pitch (2)/LConn1 -- Left Shoulder Base/RConn1
  Left Shoulder Axis/RConn1 -- Left Shoulder Pitch (2)/RConn1 -- Left Shoulder/LConn1
  Left Shoulder/RConn1 -- Left Shoulder Roll (4)/RConn1 -- Left Arm Base/RConn1
  Left Upper Arm/RConn1 -- Left Elbow (6)/LConn1 -- Left Forearm Base/RConn1
  Left Forearm Axis/RConn1 -- Left Elbow (6)/RConn1 -- Left Forearm/LConn1
  Left Arm Axis/RConn1 -- Left Shoulder Roll (4)/LConn1 -- Left Upper Arm/LConn1

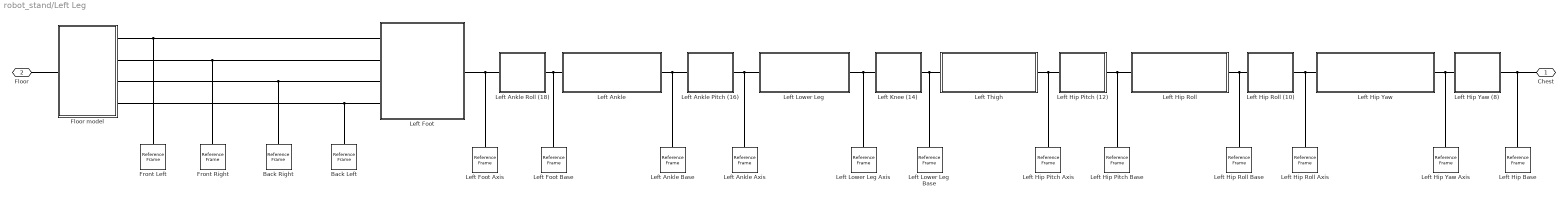
== system robot_stand/Left Leg ==
  Back Left : sm_lib/Frames and Transforms/Reference Frame  BlockFunction=simmechanics.library.frames_transforms.reference_frame
  Back Right : sm_lib/Frames and Transforms/Reference Frame  BlockFunction=simmechanics.library.frames_transforms.reference_frame
  Floor model : Subsystem
  Front Left : sm_lib/Frames and Transforms/Reference Frame  BlockFunction=simmechanics.library.frames_transforms.reference_frame
  Front Right : sm_lib/Frames and Transforms/Reference Frame  BlockFunction=simmechanics.library.frames_transforms.reference_frame
  Left Ankle : Subsystem
  Left Ankle Axis : sm_lib/Frames and Transforms/Reference Frame  BlockFunction=simmechanics.library.frames_transforms.reference_frame
  Left Ankle Base : sm_lib/Frames and Transforms/Reference Frame  BlockFunction=simmechanics.library.frames_transforms.reference_frame
  Left Ankle Pitch (16) : Subsystem
  Left Ankle Roll (18) : Subsystem
  Left Foot : Subsystem
  Left Foot Axis : sm_lib/Frames and Transforms/Reference Frame  BlockFunction=simmechanics.library.frames_transforms.reference_frame
  Left Foot Base : sm_lib/Frames and Transforms/Reference Frame  BlockFunction=simmechanics.library.frames_transforms.reference_frame
  Left Hip Base : sm_lib/Frames and Transforms/Reference Frame  BlockFunction=simmechanics.library.frames_transforms.reference_frame
  Left Hip Pitch (12) : Subsystem
  Left Hip Pitch Axis : sm_lib/Frames and Transforms/Reference Frame  BlockFunction=simmechanics.library.frames_transforms.reference_frame
  Left Hip Pitch Base : sm_lib/Frames and Transforms/Reference Frame  BlockFunction=simmechanics.library.frames_transforms.reference_frame
  Left Hip Roll : Subsystem
  Left Hip Roll (10) : Subsystem
  Left Hip Roll Axis : sm_lib/Frames and Transforms/Reference Frame  BlockFunction=simmechanics.library.frames_transforms.reference_frame
  Left Hip Roll Base : sm_lib/Frames and Transforms/Reference Frame  BlockFunction=simmechanics.library.frames_transforms.reference_frame
  Left Hip Yaw : Subsystem
  Left Hip Yaw (8) : Subsystem
  Left Hip Yaw Axis : sm_lib/Frames and Transforms/Reference Frame  BlockFunction=simmechanics.library.frames_transforms.reference_frame
  Left Knee (14) : Subsystem
  Left Lower Leg : Subsystem
  Left Lower Leg Axis : sm_lib/Frames and Transforms/Reference Frame  BlockFunction=simmechanics.library.frames_transforms.reference_frame
  Left Lower Leg Base : sm_lib/Frames and Transforms/Reference Frame  BlockFunction=simmechanics.library.frames_transforms.reference_frame
  Left Thigh : Subsystem
  Chest : PMIOPort  Port=1  Side=Right
  Floor : PMIOPort  Port=2  Side=Left
  connections:
  Chest/RConn1 -- Left Hip Yaw (8)/LConn1 -- Left Hip Base/RConn1
  Left Hip Roll/RConn1 -- Left Hip Pitch (12)/LConn1 -- Left Hip Pitch Base/RConn1
  Left Thigh/RConn1 -- Left Knee (14)/LConn1 -- Left Lower Leg Base/RConn1
  Left Lower Leg/RConn1 -- Left Ankle Pitch (16)/RConn1 -- Left Ankle Axis/RConn1
  Left Ankle/RConn1 -- Left Ankle Roll (18)/LConn1 -- Left Foot Base/RConn1
  Left Hip Yaw/LConn1 -- Left Hip Yaw (8)/RConn1 -- Left Hip Yaw Axis/RConn1
  Left Hip Roll Axis/RConn1 -- Left Hip Roll (10)/RConn1 -- Left Hip Yaw/RConn1
  Left Hip Roll Base/RConn1 -- Left Hip Roll (10)/LConn1 -- Left Hip Roll/LConn1
  Left Thigh/LConn1 -- Left Hip Pitch (12)/RConn1 -- Left Hip Pitch Axis/RConn1
  Left Lower Leg/LConn1 -- Left Knee (14)/RConn1 -- Left Lower Leg Axis/RConn1
  Left Ankle/LConn1 -- Left Ankle Pitch (16)/LConn1 -- Left Ankle Base/RConn1
  Left Foot/LConn1 -- Left Foot Axis/RConn1 -- Left Ankle Roll (18)/RConn1
  Left Foot/RConn1 -- Floor model/LConn1 -- Front Left/RConn1
  Front Right/RConn1 -- Floor model/LConn2 -- Left Foot/RConn2
  Back Right/RConn1 -- Floor model/LConn3 -- Left Foot/RConn3
  Back Left/RConn1 -- Floor model/LConn4 -- Left Foot/RConn4
  Floor/RConn1 -- Floor model/RConn1

== system robot_stand/Right Arm ==
  Right Arm Axis : sm_lib/Frames and Transforms/Reference Frame  BlockFunction=simmechanics.library.frames_transforms.reference_frame
  Right Arm Base : sm_lib/Frames and Transforms/Reference Frame  BlockFunction=simmechanics.library.frames_transforms.reference_frame
  Right Elbow (5) : Subsystem
  Right ForeArm Axis : sm_lib/Frames and Transforms/Reference Frame  BlockFunction=simmechanics.library.frames_transforms.reference_frame
  Right ForeArm Base : sm_lib/Frames and Transforms/Reference Frame  BlockFunction=simmechanics.library.frames_transforms.reference_frame
  Right Forearm : Subsystem
  Right Shoulder : Subsystem
  Right Shoulder Axis : sm_lib/Frames and Transforms/Reference Frame  BlockFunction=simmechanics.library.frames_transforms.reference_frame
  Right Shoulder Base : sm_lib/Frames and Transforms/Reference Frame  BlockFunction=simmechanics.library.frames_transforms.reference_frame
  Right Shoulder Pitch (1) : Subsystem
  Right Shoulder Roll (3) : Subsystem
  Right Upper Arm : Subsystem
  Chest : PMIOPort  Port=1  Side=Left
  connections:
  Chest/RConn1 -- Right Shoulder Pitch (1)/LConn1 -- Right Shoulder Base/RConn1
  Right Shoulder Axis/RConn1 -- Right Shoulder Pitch (1)/RConn1 -- Right Shoulder/LConn1
  Right Upper Arm/RConn1 -- Right Elbow (5)/LConn1 -- Right ForeArm Base/RConn1
  Right Arm Base/RConn1 -- Right Shoulder Roll (3)/LConn1 -- Right Shoulder/RConn1
  Right Arm Axis/RConn1 -- Right Shoulder Roll (3)/RConn1 -- Right Upper Arm/LConn1
  Right ForeArm Axis/RConn1 -- Right Elbow (5)/RConn1 -- Right Forearm/LConn1

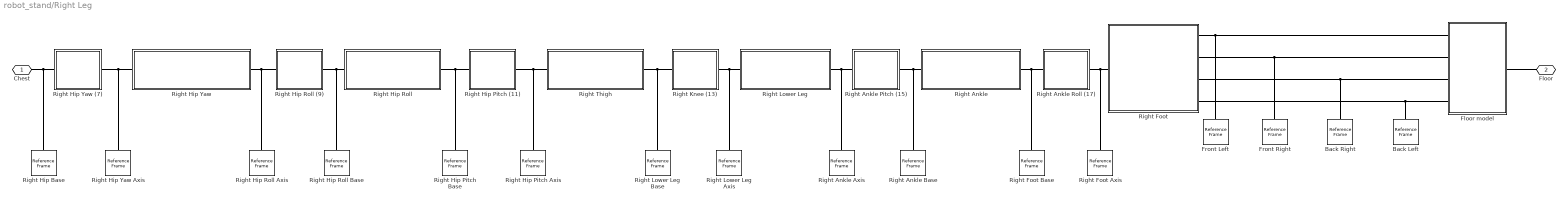
== system robot_stand/Right Leg ==
  Back Left : sm_lib/Frames and Transforms/Reference Frame  BlockFunction=simmechanics.library.frames_transforms.reference_frame
  Back Right : sm_lib/Frames and Transforms/Reference Frame  BlockFunction=simmechanics.library.frames_transforms.reference_frame
  Floor model : Subsystem
  Front Left : sm_lib/Frames and Transforms/Reference Frame  BlockFunction=simmechanics.library.frames_transforms.reference_frame
  Front Right : sm_lib/Frames and Transforms/Reference Frame  BlockFunction=simmechanics.library.frames_transforms.reference_frame
  Right Ankle : Subsystem
  Right Ankle Axis : sm_lib/Frames and Transforms/Reference Frame  BlockFunction=simmechanics.library.frames_transforms.reference_frame
  Right Ankle Base : sm_lib/Frames and Transforms/Reference Frame  BlockFunction=simmechanics.library.frames_transforms.reference_frame
  Right Ankle Pitch (15) : Subsystem
  Right Ankle Roll (17) : Subsystem
  Right Foot : Subsystem
  Right Foot Axis : sm_lib/Frames and Transforms/Reference Frame  BlockFunction=simmechanics.library.frames_transforms.reference_frame
  Right Foot Base : sm_lib/Frames and Transforms/Reference Frame  BlockFunction=simmechanics.library.frames_transforms.reference_frame
  Right Hip Base : sm_lib/Frames and Transforms/Reference Frame  BlockFunction=simmechanics.library.frames_transforms.reference_frame
  Right Hip Pitch (11) : Subsystem
  Right Hip Pitch Axis : sm_lib/Frames and Transforms/Reference Frame  BlockFunction=simmechanics.library.frames_transforms.reference_frame
  Right Hip Pitch Base : sm_lib/Frames and Transforms/Reference Frame  BlockFunction=simmechanics.library.frames_transforms.reference_frame
  Right Hip Roll : Subsystem
  Right Hip Roll (9) : Subsystem
  Right Hip Roll Axis : sm_lib/Frames and Transforms/Reference Frame  BlockFunction=simmechanics.library.frames_transforms.reference_frame
  Right Hip Roll Base : sm_lib/Frames and Transforms/Reference Frame  BlockFunction=simmechanics.library.frames_transforms.reference_frame
  Right Hip Yaw : Subsystem
  Right Hip Yaw (7) : Subsystem
  Right Hip Yaw Axis : sm_lib/Frames and Transforms/Reference Frame  BlockFunction=simmechanics.library.frames_transforms.reference_frame
  Right Knee (13) : Subsystem
  Right Lower Leg : Subsystem
  Right Lower Leg Axis : sm_lib/Frames and Transforms/Reference Frame  BlockFunction=simmechanics.library.frames_transforms.reference_frame
  Right Lower Leg Base : sm_lib/Frames and Transforms/Reference Frame  BlockFunction=simmechanics.library.frames_transforms.reference_frame
  Right Thigh : Subsystem
  Chest : PMIOPort  Port=1  Side=Left
  Floor : PMIOPort  Port=2  Side=Right
  connections:
  Chest/RConn1 -- Right Hip Yaw (7)/LConn1 -- Right Hip Base/RConn1
  Right Hip Yaw Axis/RConn1 -- Right Hip Yaw (7)/RConn1 -- Right Hip Yaw/LConn1
  Right Hip Yaw/RConn1 -- Right Hip Roll (9)/RConn1 -- Right Hip Roll Axis/RConn1
  Right Hip Roll/RConn1 -- Right Hip Pitch (11)/LConn1 -- Right Hip Pitch Base/RConn1
  Right Thigh/RConn1 -- Right Knee (13)/LConn1 -- Right Lower Leg Base/RConn1
  Right Ankle/RConn1 -- Right Ankle Roll (17)/LConn1 -- Right Foot Base/RConn1
  Right Hip Roll/LConn1 -- Right Hip Roll (9)/LConn1 -- Right Hip Roll Base/RConn1
  Right Thigh/LConn1 -- Right Hip Pitch (11)/RConn1 -- Right Hip Pitch Axis/RConn1
  Right Lower Leg/LConn1 -- Right Knee (13)/RConn1 -- Right Lower Leg Axis/RConn1
  Right Lower Leg/RConn1 -- Right Ankle Axis/RConn1 -- Right Ankle Pitch (15)/RConn1
  Right Ankle/LConn1 -- Right Ankle Pitch (15)/LConn1 -- Right Ankle Base/RConn1
  Right Foot/LConn1 -- Right Ankle Roll (17)/RConn1 -- Right Foot Axis/RConn1
  Front Left/RConn1 -- Floor model/LConn1 -- Right Foot/RConn1
  Front Right/RConn1 -- Floor model/LConn2 -- Right Foot/RConn2
  Back Right/RConn1 -- Floor model/LConn3 -- Right Foot/RConn3
  Back Left/RConn1 -- Floor model/LConn4 -- Right Foot/RConn4
  Floor model/RConn1 -- Floor/RConn1

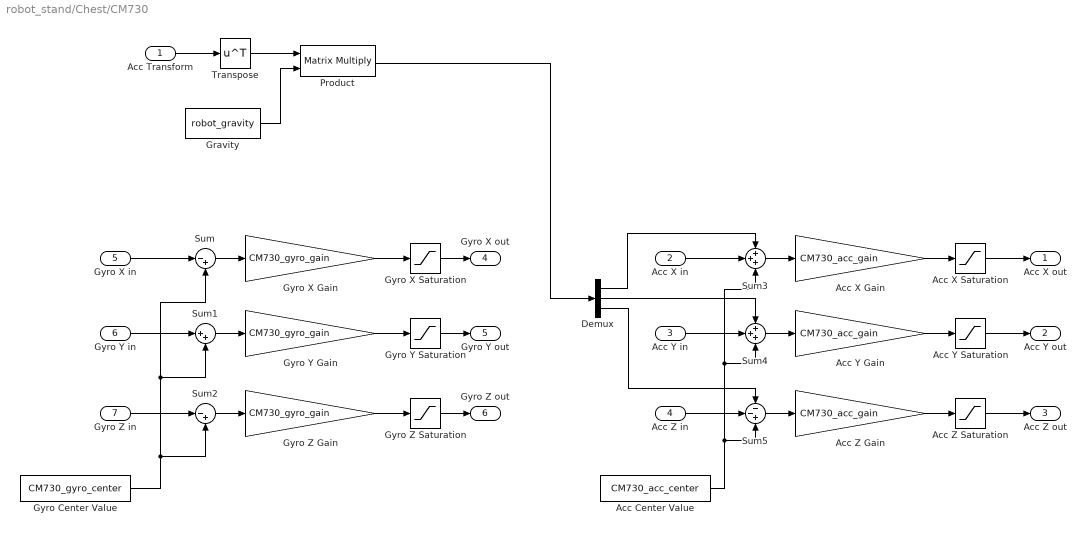
== system robot_stand/Chest/CM730 ==
  Acc Transform : Inport
  Acc X in : Inport  Port=2
  Acc Y in : Inport  Port=3
  Acc Z in : Inport  Port=4
  Gyro X in : Inport  Port=5
  Gyro Y in : Inport  Port=6
  Gyro Z in : Inport  Port=7
  Acc Center Value : Constant  Value=CM730_acc_center
  Acc X Gain : Gain  Gain=CM730_acc_gain  OutMax=1023  OutDataTypeStr=int16  SaturateOnIntegerOverflow=on
  Acc X Saturation : Saturate  UpperLimit=1023  LowerLimit=0
  Acc Y Gain : Gain  Gain=CM730_acc_gain  OutDataTypeStr=int16  SaturateOnIntegerOverflow=on
  Acc Y Saturation : Saturate  UpperLimit=1023  LowerLimit=0
  Acc Z Gain : Gain  Gain=CM730_acc_gain  OutDataTypeStr=int16  SaturateOnIntegerOverflow=on
  Acc Z Saturation : Saturate  UpperLimit=1023  LowerLimit=0
  Demux : Demux  Outputs=3
  Gravity : Constant  Value=robot_gravity
  Gyro Center Value : Constant  Value=CM730_gyro_center
  Gyro X Gain : Gain  Gain=CM730_gyro_gain  OutDataTypeStr=int16  SaturateOnIntegerOverflow=on
  Gyro X Saturation : Saturate  UpperLimit=1023  LowerLimit=0
  Gyro Y Gain : Gain  Gain=CM730_gyro_gain  OutDataTypeStr=int16  SaturateOnIntegerOverflow=on
  Gyro Y Saturation : Saturate  UpperLimit=1023  LowerLimit=0
  Gyro Z Gain : Gain  Gain=CM730_gyro_gain  OutDataTypeStr=int16  SaturateOnIntegerOverflow=on
  Gyro Z Saturation : Saturate  UpperLimit=1023  LowerLimit=0
  Product : Product  Multiplication=Matrix(*)
  Sum : Sum  Inputs=|-+
  Sum1 : Sum  Inputs=|++
  Sum2 : Sum  Inputs=|-+
  Sum3 : Sum  Inputs=+++
  Sum4 : Sum  Inputs=+++
  Sum5 : Sum  Inputs=--+
  Transpose : Math  Operator=transpose  SaturateOnIntegerOverflow=on
  Acc X out : Outport
  Acc Y out : Outport  Port=2
  Acc Z out : Outport  Port=3
  Gyro X out : Outport  Port=4
  Gyro Y out : Outport  Port=5
  Gyro Z out : Outport  Port=6
  wires:
  Gyro X Gain/1 -> Gyro X Saturation/1
  Gyro Y Gain/1 -> Gyro Y Saturation/1
  Product/1 -> Demux/1
  Acc X Gain/1 -> Acc X Saturation/1
  Acc Y Gain/1 -> Acc Y Saturation/1
  Acc Z Gain/1 -> Acc Z Saturation/1
  Sum/1 -> Gyro X Gain/1
  Gyro X in/1 -> Sum/1
  Sum2/1 -> Gyro Z Gain/1
  Gyro Z in/1 -> Sum2/1
  Gyro Y in/1 -> Sum1/1
  Sum1/1 -> Gyro Y Gain/1
  Gyro Center Value/1 -> Sum2/2, Sum1/2, Sum/2
  Sum3/1 -> Acc X Gain/1
  Acc X in/1 -> Sum3/2
  Acc Y in/1 -> Sum4/2
  Sum4/1 -> Acc Y Gain/1
  Sum5/1 -> Acc Z Gain/1
  Acc Z in/1 -> Sum5/2
  Acc Center Value/1 -> Sum5/3, Sum4/3, Sum3/3
  Demux/1 -> Sum3/1
  Demux/2 -> Sum4/1
  Demux/3 -> Sum5/1
  Gyro Z Gain/1 -> Gyro Z Saturation/1
  Acc Transform/1 -> Transpose/1
  Gravity/1 -> Product/2
  Transpose/1 -> Product/1
  Gyro X Saturation/1 -> Gyro X out/1
  Gyro Y Saturation/1 -> Gyro Y out/1
  Gyro Z Saturation/1 -> Gyro Z out/1
  Acc X Saturation/1 -> Acc X out/1
  Acc Y Saturation/1 -> Acc Y out/1
  Acc Z Saturation/1 -> Acc Z out/1

== system robot_stand/Head/Head ==
  Solid : sm_lib/Body Elements/Solid  InertiaType=Custom  Mass=137.28  MassUnits=g  CenterOfMass=[-18.87 -0.74 24.23]  CenterOfMassUnits=mm  MomentsOfInertia=[89712 78117 81581]  MomentsOfInertiaUnits=g*mm^2  ProductsOfInertia=[-47.47 665.61 10975]  ProductsOfInertiaUnits=g*mm^2  DensityBased=on  Density=1000  DensityUnits=kg/(m^3)  GraphicType=FromGeometry  MarkerShape=Sphere  MarkerSize=10  MarkerSizeUnits=m  GraphicVisPropType=SimpleVisualProperties  GraphicDiffuseColor=[0.5 0.5 0.5]  GraphicSpecularColor=[0.5 0.5 0.5 1.0]  GraphicAmbientColor=[0.15 0.15 0.15 1.0]  GraphicEmissiveColor=[0.0 0.0 0.0 1.0]  GraphicShininess=75  GraphicOpacity=1.0  GeometryShape=FromFile  RectangleSize=[1 1]  RectangleSizeUnits=m  BrickDimensions=[1 1 1]  BrickDimensionUnits=m  CylinderRadius=1  CylinderRadiusUnits=m  CylinderLength=1  CylinderLengthUnits=m  SphereRadius=1  SphereRadiusUnits=m  EllipsoidRadii=[1 1 1]  EllipsoidRadiiUnits=m  ExtrusionCrossSection=[1 1; -1 1; -1 -1; 1 -1]  ExtrusionCrossSectionUnits=m  ExtrusionLength=1  ExtrusionLengthUnits=m  PolygonNumSides=3  PolygonOuterRadius=1  PolygonOuterRadiusUnits=m  ExtGeomFileType=STL  ExtGeomFileName=D:\Ker Lann\systemes\darwin\kinematics\STL\Head.STL  ExtGeomFileUnits=mm  RevolutionCrossSection=[1 1; 1 -1; 2 -1; 2 1]  RevolutionCrossSectionUnits=m  RevolutionExtent=Full  RevolutionAngle=180  RevolutionAngleUnits=deg  BlockFunction=simmechanics.library.body_elements.solid
  Head Tilt : PMIOPort  Port=1  Side=Left
  connections:
  Head Tilt/RConn1 -- Solid/RConn1
